simulink model "linear_system_avec_controleur"  (R2021b)
settings: Solver=VariableStepAuto  StartTime=0.0  StopTime=200  RelTol=1e-3
values from neighbouring files (symbols this model uses):
  A = [0 0 0  1 0 0   0 0 0   0 0 0 ... (first row only)    [systune_constant_gain_LPV.m]    (also in systune_gain_scheduling.m; systune_variable_gain_scheduling_LPV.m)
  B = diag([ws; chord; ws])    [external_force_moment.m]    (also in systune_constant_gain_LPV.m = [0 0 0 0; systune_gain_scheduling.m = [0 0 0 0; systune_variable_gain_scheduling_LPV.m = [0 0 0 0)
  B2 = [0 0 ... (first row only)    [systune_constant_gain_LPV.m]    (also in systune_gain_scheduling.m; systune_variable_gain_scheduling_LPV.m)
  H_val = [0.174893532101 -0.170983587428 0.116298770163 -0.120491253945 -0.591123259979 0.466999830321 0.606251408925 -0.36729072329 0.527922365719 -0.579504209683 -0.860165616929 0.217648206511 ... (22 elements, 2x11)]    [matrix.mat]    (also in systune_constant_gain_LPV.m = H_val.D; systune_gain_scheduling.m = H_val.D; systune_variable_gain_scheduling_LPV.m = getBlockValue(T,'H'))
  K_val = [-0.717823721707 -0.535586914826 0.293461018845 0.259857970212 -0.116645066118 0.0068635572033 0.0510701432383 0.0105656377564 -0.103136434688 -0.470758687236 -0.215457393556 0.229494669048 ... (44 elements, 4x11)]    [matrix.mat]    (also in systune_constant_gain_LPV.m = K_val.D; systune_gain_scheduling.m = K_val.D; systune_variable_gain_scheduling_LPV.m = getBlockValue(T,'K'))
  u_eq = [2.43630788633 2.43630788633 0 0]    [matrix.mat]    (also in matrix_lqr.mat = [1.98073811897 1.98073811897 0 0]; systune_constant_gain_LPV.m = [ua;ua;ub;ub]; systune_gain_scheduling.m = [ua;ua;ub;ub]; systune_variable_gain_scheduling_LPV.m = [ua;ua;ub;ub])
  w = [-i*0.4;0;0]    [systune_constant_gain_LPV.m]    (also in systune_gain_scheduling.m = [0;0;0]; systune_variable_gain_scheduling_LPV.m = [-i;0;0])
  x_12 = [[0; 0; 0]; [0; 0; 0]; [0; sin(angle/2); 0]; [0; 0; 0]]    [systune_constant_gain_LPV.m]    (also in systune_gain_scheduling.m; systune_variable_gain_scheduling_LPV.m)
settings Model: Creator=florian  LastModifiedBy=florian

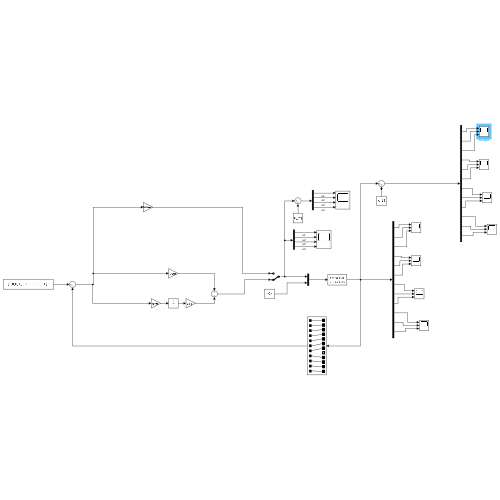
[thumbnail: Simulink's stored preview of the top-level diagram]
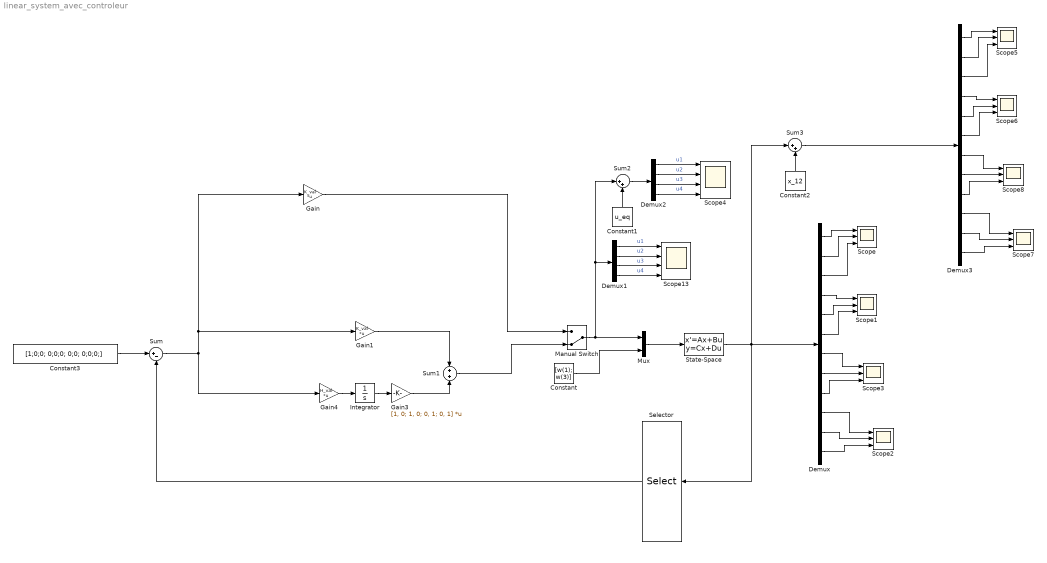
== system linear_system_avec_controleur ==
  Constant : Constant  Value=[w(1); w(3)]
  Constant1 : Constant  Value=u_eq  VectorParams1D=off
  Constant2 : Constant  Value=x_12  VectorParams1D=off
  Constant3 : Constant  Value=[1;0;0; 0;0;0; 0;0; 0;0;0;]
  Demux : Demux  Outputs=12
  Demux1 : Demux
  Demux2 : Demux
  Demux3 : Demux  Outputs=12
  Gain : Gain  Gain=K_val  Multiplication=Matrix(K*u) (u vector)
  Gain1 : Gain  Gain=K_val  Multiplication=Matrix(K*u) (u vector)
  Gain3 : Gain  Gain=[1, 0; 1, 0; 0, 1; 0, 1]  Multiplication=Matrix(K*u) (u vector)
  Gain4 : Gain  Gain=H_val  Multiplication=Matrix(K*u) (u vector)
  Integrator : Integrator  InitialCondition=zeros(1,2)
  Manual Switch : ManualSwitch  CurrentSetting=0
  Mux : Mux  Inputs=2
  Scope{,1..3,5..8} (8 alike) : Scope  NumInputPorts=3
  Scope13 : Scope  NumInputPorts=4
  Scope4 : Scope  NumInputPorts=4
  Selector : Selector  InputPortWidth=12  IndexOptions=Index vector (dialog)  Indices=[1:7 9:12]  OutputSizes=1
  State-Space : StateSpace  A=A  B=[B, B2]  C=eye(12)  D=zeros(12,6)  InitialCondition=zeros(12,1)
  Sum : Sum  Inputs=|+-
  Sum1 : Sum
  Sum2 : Sum  Inputs=|++
  Sum3 : Sum  Inputs=|++
  wires:
  Mux/1 -> State-Space/1
  Constant3/1 -> Sum/1
  Sum/1 -> Gain4/1, Gain1/1, Gain/1
  Demux/1 -> Scope/1
  Demux/2 -> Scope/2
  Demux/3 -> Scope/3
  Demux/4 -> Scope1/1
  Demux/5 -> Scope1/2
  Demux/6 -> Scope1/3
  Gain4/1 -> Integrator/1
  Integrator/1 -> Gain3/1
  Gain3/1 -> Sum1/2
  Gain1/1 -> Sum1/1
  Sum1/1 -> Manual Switch/2
  Gain/1 -> Manual Switch/1
  Demux1/4 -> Scope13/4  "u4"
  Demux1/3 -> Scope13/3  "u3"
  Demux1/1 -> Scope13/1  "u1"
  Demux1/2 -> Scope13/2  "u2"
  Selector/1 -> Sum/2
  Demux/12 -> Scope2/3
  Demux/11 -> Scope2/2
  Demux/10 -> Scope2/1
  Demux/7 -> Scope3/1
  Demux/8 -> Scope3/2
  Demux/9 -> Scope3/3
  Manual Switch/1 -> Demux1/1, Sum2/1, Mux/1
  Constant1/1 -> Sum2/2
  Demux2/4 -> Scope4/4  "u4"
  Demux2/1 -> Scope4/1  "u1"
  Sum2/1 -> Demux2/1
  Demux2/3 -> Scope4/3  "u3"
  Demux2/2 -> Scope4/2  "u2"
  Constant2/1 -> Sum3/2
  State-Space/1 -> Sum3/1, Selector/1, Demux/1
  Demux3/8 -> Scope8/2
  Demux3/6 -> Scope6/3
  Demux3/4 -> Scope6/1
  Demux3/3 -> Scope5/3
  Demux3/9 -> Scope8/3
  Sum3/1 -> Demux3/1
  Demux3/5 -> Scope6/2
  Demux3/1 -> Scope5/1
  Demux3/10 -> Scope7/1
  Demux3/12 -> Scope7/3
  Demux3/7 -> Scope8/1
  Demux3/2 -> Scope5/2
  Demux3/11 -> Scope7/2
  Constant/1 -> Mux/2
